simulink model "fuel_cell_characteristic"  (R2021a)
settings: Solver=VariableStepAuto  StartTime=0.001  StopTime=460  RelTol=1e-3
libraries: simulink x1
settings Model: Creator=Admin  LastModifiedBy=Admin

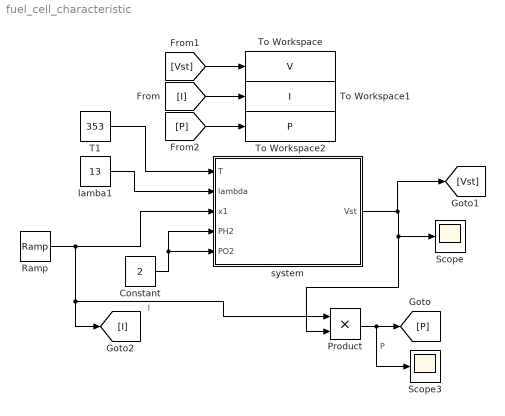
== system fuel_cell_characteristic ==
  Constant : Constant  Value=2
  Product : Product
  Ramp : simulink/Sources/Ramp  slope=1  start=0  InitialOutput=0
  Scope : Scope
  Scope3 : Scope
  T1 : Constant  Value=353
  To Workspace : ToWorkspace  VariableName=V  SampleTime=0.05
      settings: Decimation=2
  To Workspace1 : ToWorkspace  VariableName=I  SampleTime=0.05
      settings: Decimation=2
  To Workspace2 : ToWorkspace  VariableName=P  SampleTime=0.05
      settings: Decimation=2
  lamba1 : Constant  Value=13
  system : MATLAB Function  TreatAsAtomicUnit=on
  wires:
  Constant/1 -> system/4(PH2), system/5(PO2)
  T1/1 -> system/1(T)
  lamba1/1 -> system/2(lambda)
  Ramp/1 -> [I], Product/1, system/3(x1)  "I"
  system/1(Vst) -> Product/2, Scope/1, [Vst]
  Product/1 -> Scope3/1, [P]  "P"
  [Vst] -> To Workspace/1
  [I] -> To Workspace1/1
  [P] -> To Workspace2/1

== matlab function fuel_cell_characteristic/system ==
  data: T input; lambda input; x1 input; Vst output; PH2 input; PO2 input
function Vst = circuit(T,lambda,x1,PH2,PO2)
N = 24;
A = 232;
m1 = 0.944;
m2 = -0.00354; 
m3 = -7.8*10^-8;
m4 = 1.96*10^-4;
n = 2;
iL = 2; 
R = 83144.7; 
F = 96484600;
CO2 = PO2/((5.08*10^6)*exp(-498/T));
rm = (181.6*(1+0.03*(x1/A)+0.062*((T/303)^2)*(x1/A)^2.5))/((lambda-0.634-3*x1/A)*exp(4.18*(T-303/T))); 
tm = 175*10^-4;
Rm = rm*tm/A;
E = 1.229-8.5*(10^-4)*(T-298.15)+4.308*(10^-5)*T*(log(PH2)+log(PO2));
Vact = m1+m2*T+m3*T*log(CO2)+m4*T*log(x1);
Vohmic = x1*Rm;
Vcon = (-R*T/(n*F))*log(1-x1/(iL*A));
Vcell = E - Vact - Vohmic - Vcon;
Vst = N*Vcell;
